simulink model "CP_ContrSys_NLin_n9558292"  (R2018a)
settings: Solver=VariableStepAuto  StartTime=0.0  StopTime=10.0  RelTol=1e-3
values from neighbouring files (symbols this model uses):
  Aa = [0,0,1,0;0,0,0,1;0,-m*g/Mc,0,0;0,g*(Mc+m)/(l*Mc),0,0]    [CP_ContrSys_Lin_a_MainFile_n9558292.m]    (also in CP_ContrSys_Lin_b_MainFile_n9558292.m = [0,0,1,0;0,0,0,1;0,-m*g/Mc,0,0;0,-g*(Mc+m)/(l*Mc),0,0])
  Ba = [0;0;1/Mc;-1/(l*Mc)]    [CP_ContrSys_Lin_a_MainFile_n9558292.m]    (also in CP_ContrSys_Lin_b_MainFile_n9558292.m = [0;0;1/Mc;1/(l*Mc)])
  Ca = [1,0,0,0;0,1,0,0]    [CP_ContrSys_Lin_a_MainFile_n9558292.m]    (also in CP_ContrSys_Lin_b_MainFile_n9558292.m)
  g = 9.81    [CP_ContrSys_Lin_a_MainFile_n9558292.m]    (also in CP_ContrSys_Lin_b_MainFile_n9558292.m)
  K_SF = Ka    [CP_ContrSys_Lin_a_MainFile_n9558292.m]    (also in CP_ContrSys_Lin_b_MainFile_n9558292.m)
  l = 0.2    [CP_ContrSys_Lin_a_MainFile_n9558292.m]    (also in CP_ContrSys_Lin_b_MainFile_n9558292.m)
  La = place(Aa',Ca',PLa)'    [CP_ContrSys_Lin_a_MainFile_n9558292.m]    (also in CP_ContrSys_Lin_b_MainFile_n9558292.m)
  m = 0.15    [CP_ContrSys_Lin_a_MainFile_n9558292.m]    (also in CP_ContrSys_Lin_b_MainFile_n9558292.m)
  Mc = 0.4    [CP_ContrSys_Lin_a_MainFile_n9558292.m]    (also in CP_ContrSys_Lin_b_MainFile_n9558292.m)
  x10 = 0.2    [CP_ContrSys_Lin_a_MainFile_n9558292.m]    (also in CP_ContrSys_Lin_b_MainFile_n9558292.m)
  x1_bar = 0    [CP_ContrSys_Lin_a_MainFile_n9558292.m]    (also in CP_ContrSys_Lin_b_MainFile_n9558292.m)
  x20 = deg2rad(20)    [CP_ContrSys_Lin_a_MainFile_n9558292.m]    (also in CP_ContrSys_Lin_b_MainFile_n9558292.m = deg2rad(200))
  x2_bar = 0    [CP_ContrSys_Lin_a_MainFile_n9558292.m]    (also in CP_ContrSys_Lin_b_MainFile_n9558292.m = 3.14159265359)
  x30 = 0    [CP_ContrSys_Lin_a_MainFile_n9558292.m]    (also in CP_ContrSys_Lin_b_MainFile_n9558292.m)
  x40 = 0    [CP_ContrSys_Lin_a_MainFile_n9558292.m]    (also in CP_ContrSys_Lin_b_MainFile_n9558292.m)
settings Model: Creator=haidarobeid  LastModifiedBy=haidarobeid

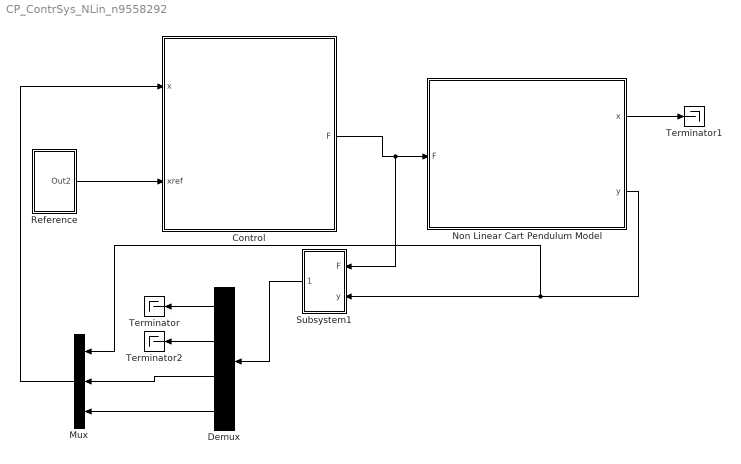
== system CP_ContrSys_NLin_n9558292 ==
  Control : Subsystem
  Demux : Demux
  Mux : Mux  Inputs=3
  Non Linear Cart Pendulum Model : Subsystem
  Reference : Subsystem
  Subsystem1 : Subsystem
  Terminator : Terminator
  Terminator1 : Terminator
  Terminator2 : Terminator
  wires:
  Non Linear Cart Pendulum Model/2(y) -> Mux/1, Subsystem1/2(y)
  Reference/1(Out2) -> Control/2(xref)
  Control/1("F ") -> Subsystem1/1(F), Non Linear Cart Pendulum Model/1(F)
  Demux/1 -> Terminator/1
  Demux/3 -> Mux/2
  Subsystem1/1(xhat) -> Demux/1
  Demux/2 -> Terminator2/1
  Demux/4 -> Mux/3
  Non Linear Cart Pendulum Model/1(x) -> Terminator1/1
  Mux/1 -> Control/1(x)

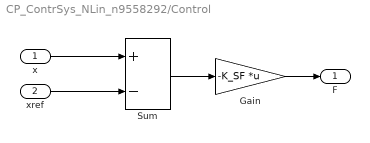
== system CP_ContrSys_NLin_n9558292/Control ==
  x : Inport
  xref : Inport  Port=2
  Gain : Gain  Gain=-K_SF  Multiplication=Matrix(K*u)
  Sum : Sum  Inputs=+-
  "F " : Outport
  wires:
  xref/1 -> Sum/2
  Gain/1 -> "F "/1
  x/1 -> Sum/1
  Sum/1 -> Gain/1

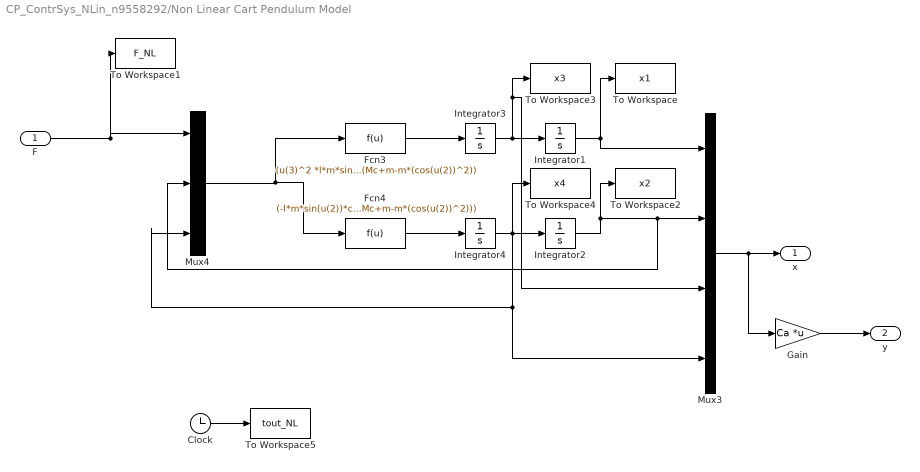
== system CP_ContrSys_NLin_n9558292/Non Linear Cart Pendulum Model ==
  F : Inport
  Clock : Clock
  Fcn3 : Fcn  Expr=(u(3)^2 *l*m*sin(u(2)) - g*m*sin(u(2))*cos(u(2)) +u(1))/(Mc+m-m*(cos(u(2))^2))
  Fcn4 : Fcn  Expr=(-l*m*sin(u(2))*cos(u(2))*u(3)^2 + g*(Mc+m)*sin(u(2)) - cos(u(2))*u(1) )/(l*(Mc+m-m*(cos(u(2))^2)))
  Gain : Gain  Gain=Ca  Multiplication=Matrix(K*u)
  Integrator1 : Integrator  InitialCondition=x10
  Integrator2 : Integrator  InitialCondition=x20
  Integrator3 : Integrator  InitialCondition=x30
  Integrator4 : Integrator  InitialCondition=x40
  Mux3 : Mux
  Mux4 : Mux  Inputs=3
  To Workspace : ToWorkspace  VariableName=x1  SampleTime=-1
  To Workspace1 : ToWorkspace  VariableName=F_NL  SampleTime=-1
  To Workspace2 : ToWorkspace  VariableName=x2  SampleTime=-1
  To Workspace3 : ToWorkspace  VariableName=x3  SampleTime=-1
  To Workspace4 : ToWorkspace  VariableName=x4  SampleTime=-1
  To Workspace5 : ToWorkspace  VariableName=tout_NL  SampleTime=-1
  x : Outport
  y : Outport  Port=2
  wires:
  Fcn3/1 -> Integrator3/1
  Fcn4/1 -> Integrator4/1
  Mux3/1 -> Gain/1, x/1
  Integrator4/1 -> Mux4/3, Mux3/4, Integrator2/1, To Workspace4/1
  Integrator2/1 -> To Workspace2/1, Mux4/2, Mux3/2
  F/1 -> To Workspace1/1, Mux4/1
  Integrator1/1 -> Mux3/1, To Workspace/1
  Integrator3/1 -> Integrator1/1, Mux3/3, To Workspace3/1
  Mux4/1 -> Fcn4/1, Fcn3/1
  Clock/1 -> To Workspace5/1
  Gain/1 -> y/1

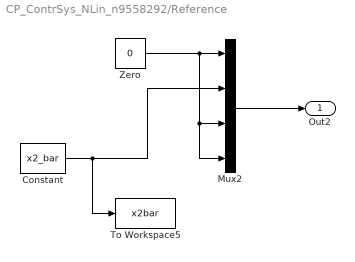
== system CP_ContrSys_NLin_n9558292/Reference ==
  Constant : Constant  Value=x2_bar
  Mux2 : Mux
  To Workspace5 : ToWorkspace  VariableName=x2bar  SaveFormat=Timeseries  SampleTime=-1
  Zero : Constant  Value=0
  Out2 : Outport
  wires:
  Mux2/1 -> Out2/1
  Constant/1 -> To Workspace5/1, Mux2/2
  Zero/1 -> Mux2/4, Mux2/3, Mux2/1

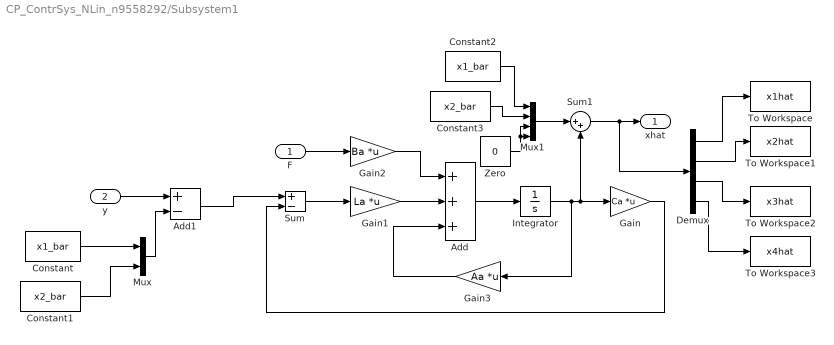
== system CP_ContrSys_NLin_n9558292/Subsystem1 ==
  F : Inport
  y : Inport  Port=2
  Add : Sum  Inputs=+++
  Add1 : Sum  Inputs=+-
  Constant : Constant  Value=x1_bar
  Constant1 : Constant  Value=x2_bar
  Constant2 : Constant  Value=x1_bar
  Constant3 : Constant  Value=x2_bar
  Demux : Demux
  Gain : Gain  Gain=Ca  Multiplication=Matrix(K*u)
  Gain1 : Gain  Gain=La  Multiplication=Matrix(K*u)
  Gain2 : Gain  Gain=Ba  Multiplication=Matrix(K*u)
  Gain3 : Gain  Gain=Aa  Multiplication=Matrix(K*u)
  Integrator : Integrator
  Mux : Mux  Inputs=2
  Mux1 : Mux
  Sum : Sum  Inputs=+-
  Sum1 : Sum  Inputs=|++
  To Workspace : ToWorkspace  VariableName=x1hat  SampleTime=-1
  To Workspace1 : ToWorkspace  VariableName=x2hat  SampleTime=-1
  To Workspace2 : ToWorkspace  VariableName=x3hat  SampleTime=-1
  To Workspace3 : ToWorkspace  VariableName=x4hat  SampleTime=-1
  Zero : Constant  Value=0
  xhat : Outport
  wires:
  Demux/1 -> To Workspace/1
  Demux/3 -> To Workspace2/1
  Gain2/1 -> Add/1
  Integrator/1 -> Sum1/2, Gain/1, Gain3/1
  Gain1/1 -> Add/2
  Add/1 -> Integrator/1
  Gain3/1 -> Add/3
  Sum/1 -> Gain1/1
  Demux/2 -> To Workspace1/1
  Gain/1 -> Sum/2
  F/1 -> Gain2/1
  Demux/4 -> To Workspace3/1
  y/1 -> Add1/1
  Add1/1 -> Sum/1
  Mux/1 -> Add1/2
  Constant/1 -> Mux/1
  Constant1/1 -> Mux/2
  Sum1/1 -> Demux/1, xhat/1
  Mux1/1 -> Sum1/1
  Constant2/1 -> Mux1/1
  Constant3/1 -> Mux1/2
  Zero/1 -> Mux1/4, Mux1/3
